simulink model "uas_main"  (R2022a)
settings: Solver=FixedStepAuto  StartTime=0.0  StopTime=10  FixedStep=sample_time  RelTol=1e-3
model workspace: external: MAT-File (data not in the file)
values from neighbouring files (symbols this model uses):
  arm_length = 0.17    [uas_trajectory.m]
  drag_coefficient = 0.47    [uas_trajectory.m]
  g = 9.80665    [uas_trajectory.m]
  inertia_xx = 0.007    [uas_trajectory.m]
  inertia_yy = 0.007    [uas_trajectory.m]
  inertia_zz = 0.012    [uas_trajectory.m]
  mass_drone = 0.68    [uas_trajectory.m]
  mass_total = mass_drone + mass_rod + mass_tip    (= 0.68)    [uas_trajectory.m]
  max_rot_velocity = 838    [uas_trajectory.m]
  mix_matrix = inv(motor_constant * allocation_matrix)    [uas_trajectory.m]
  moment_constant = 0.016    [uas_trajectory.m]
  motor_constant = 8.54858e-06    [uas_trajectory.m]
  poly_traj = uas_minimum_snap(knots, order, waypoints, corridors, make_plots)    [uas_trajectory.m]
  publish_rate = 1 * sample_time    (= 0.04)    [uas_trajectory.m]
  reference_area = pi * 75e-3^2    (= 0.0176714586764)    [uas_trajectory.m]
  rotor_offset_top = 0.01    [uas_trajectory.m]
  route = [0 0 1 ; 9 0 1 ; 9 9 1]    [uas_trajectory.m]
  sample_time = 4e-2    (= 0.04)    [uas_trajectory.m]
  x0 = 36    [uas_trajectory.m]
  y0 = 80    [uas_trajectory.m]
  z0 = 1    [uas_trajectory.m]
undefined symbols (not defined in the file or in its folder): Angular, Linear, Pose, Position, quat2rotm, X, Y, Z
libraries: nesl_utility x32, sm_lib x25, robotlib x9, simulink x1, sim3dlib x1, uavsim3dlib x1, vrlib x1
(part 2 of 2)

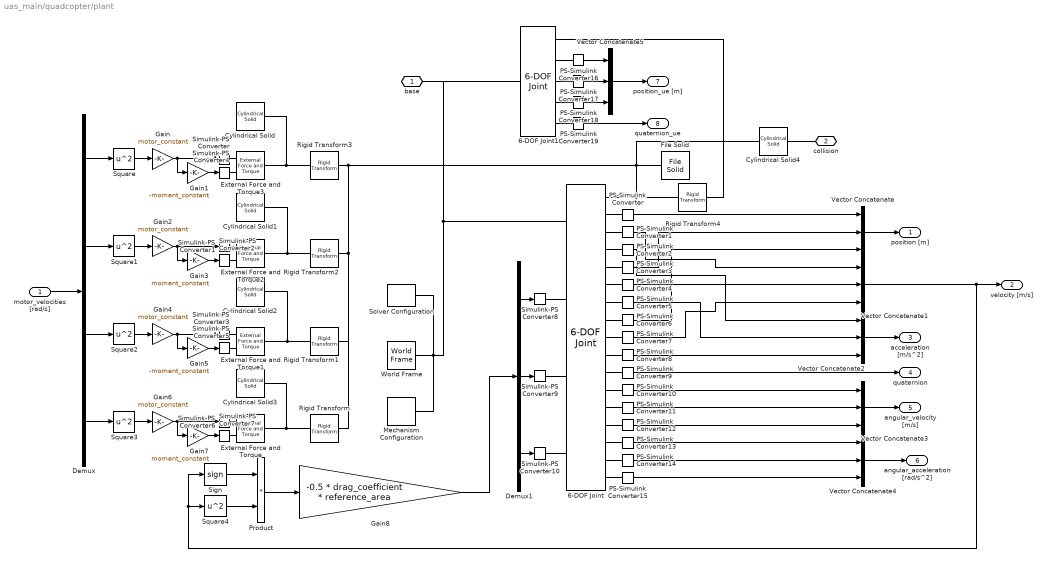
== system uas_main/quadcopter/plant ==
  motor_velocities [rad/s] : Inport
  6-DOF Joint : sm_lib/Joints/6-DOF Joint  JointMode=Normal  SenseConstraintForce=off  SenseConstraintForceX=off  SenseConstraintForceY=off  SenseConstraintForceZ=off  SenseConstraintTorque=off  SenseConstraintTorqueX=off  SenseConstraintTorqueY=off  SenseConstraintTorqueZ=off  SenseTotalForce=off  SenseTotalForceX=off  SenseTotalForceY=off  SenseTotalForceZ=off  SenseTotalTorque=off  SenseTotalTorqueX=off  SenseTotalTorqueY=off  SenseTotalTorqueZ=off  CompositeWrenchDir=BaseOnFollower  CompositeWrenchFrame=BaseFrame  PxEquilibriumPosition=0  PxEquilibriumPositionUnits=m  PxSpringStiffness=0  PxSpringStiffnessUnits=N/m  PxDampingCoefficient=0  PxDampingCoefficientUnits=N/(m/s)  PxTorqueActuationMode=InputTorque  PxMotionActuationMode=ComputedMotion  PxSensePosition=on  PxSenseVelocity=on  PxSenseAcceleration=on  PxSenseTorqueForce=off  PxSenseLowerLimitTorqueForce=off  PxSenseUpperLimitTorqueForce=off  PxLowerLimitSpecify=off  PxLowerLimitBound=-1  PxLowerLimitBoundUnits=m  PxLowerLimitStiffness=1e6  PxLowerLimitStiffnessUnits=N/m  PxLowerLimitDamping=1e3  PxLowerLimitDampingUnits=N/(m/s)  PxLowerLimitTransitionRegionWidth=1e-4  PxLowerLimitTransitionRegionWidthUnits=m  PxUpperLimitSpecify=off  PxUpperLimitBound=1  PxUpperLimitBoundUnits=m  PxUpperLimitStiffness=1e6  PxUpperLimitStiffnessUnits=N/m  PxUpperLimitDamping=1e3  PxUpperLimitDampingUnits=N/(m/s)  PxUpperLimitTransitionRegionWidth=1e-4  PxUpperLimitTransitionRegionWidthUnits=m  PxPositionTargetSpecify=on  PxPositionTargetPriority=High  PxPositionTargetValue=0  PxPositionTargetValueUnits=m  PxVelocityTargetSpecify=off  PxVelocityTargetPriority=High  PxVelocityTargetValue=0  PxVelocityTargetValueUnits=m/s  PyEquilibriumPosition=0  PyEquilibriumPositionUnits=m  PySpringStiffness=0  PySpringStiffnessUnits=N/m  PyDampingCoefficient=0  PyDampingCoefficientUnits=N/(m/s)  PyTorqueActuationMode=InputTorque  PyMotionActuationMode=ComputedMotion  PySensePosition=on  PySenseVelocity=on  PySenseAcceleration=on  PySenseTorqueForce=off  PySenseLowerLimitTorqueForce=off  PySenseUpperLimitTorqueForce=off  PyLowerLimitSpecify=off  PyLowerLimitBound=-1  PyLowerLimitBoundUnits=m  PyLowerLimitStiffness=1e6  PyLowerLimitStiffnessUnits=N/m  PyLowerLimitDamping=1e3  PyLowerLimitDampingUnits=N/(m/s)  PyLowerLimitTransitionRegionWidth=1e-4  PyLowerLimitTransitionRegionWidthUnits=m  PyUpperLimitSpecify=off  PyUpperLimitBound=1  PyUpperLimitBoundUnits=m  PyUpperLimitStiffness=1e6  PyUpperLimitStiffnessUnits=N/m  PyUpperLimitDamping=1e3  PyUpperLimitDampingUnits=N/(m/s)  PyUpperLimitTransitionRegionWidth=1e-4  PyUpperLimitTransitionRegionWidthUnits=m  PyPositionTargetSpecify=on  PyPositionTargetPriority=High  PyPositionTargetValue=0  PyPositionTargetValueUnits=m  PyVelocityTargetSpecify=off  PyVelocityTargetPriority=High  PyVelocityTargetValue=0  PyVelocityTargetValueUnits=m/s  PzEquilibriumPosition=0  PzEquilibriumPositionUnits=m  PzSpringStiffness=0  PzSpringStiffnessUnits=N/m  PzDampingCoefficient=0  PzDampingCoefficientUnits=N/(m/s)  PzTorqueActuationMode=InputTorque  PzMotionActuationMode=ComputedMotion  PzSensePosition=on  PzSenseVelocity=on  PzSenseAcceleration=on  PzSenseTorqueForce=off  PzSenseLowerLimitTorqueForce=off  PzSenseUpperLimitTorqueForce=off  PzLowerLimitSpecify=off  PzLowerLimitBound=-1  PzLowerLimitBoundUnits=m  PzLowerLimitStiffness=1e6  PzLowerLimitStiffnessUnits=N/m  PzLowerLimitDamping=1e3  PzLowerLimitDampingUnits=N/(m/s)  PzLowerLimitTransitionRegionWidth=1e-4  PzLowerLimitTransitionRegionWidthUnits=m  PzUpperLimitSpecify=off  PzUpperLimitBound=1  PzUpperLimitBoundUnits=m  PzUpperLimitStiffness=1e6  PzUpperLimitStiffnessUnits=N/m  PzUpperLimitDamping=1e3  PzUpperLimitDampingUnits=N/(m/s)  PzUpperLimitTransitionRegionWidth=1e-4  PzUpperLimitTransitionRegionWidthUnits=m  PzPositionTargetSpecify=on  PzPositionTargetPriority=High  PzPositionTargetValue=z0  PzPositionTargetValueUnits=m  PzVelocityTargetSpecify=off  PzVelocityTargetPriority=High  PzVelocityTargetValue=0  PzVelocityTargetValueUnits=m/s  SphDefPosRotationMethod=None  SphDefPosRotationAngleUnits=deg  SphDefPosRotationStandardAxis=+Z  SphDefPosRotationAngle=0.0  SphDefPosRotationArbitraryAxis=[0 0 1]  SphDefPosFollAlignAxisA=+X  SphDefPosBaseAlignAxisA=+Y  SphDefPosFollAlignAxisB=+Y  SphDefPosBaseAlignAxisB=+Z  SphDefPosRotationSequenceAxes=FollowerAxes  SphDefPosRotationSequence=XYX  SphDefPosRotationSequenceAngles=[0 0 0]  SphDefPosRotationSequenceAnglesUnits=deg  SphDefPosRotationMatrix=[1 0 0; 0 1 0; 0 0 1]  SphEqPosRotationMethod=None  SphEqPosRotationAngleUnits=deg  SphEqPosRotationStandardAxis=+Z  SphEqPosRotationAngle=0.0  SphEqPosRotationArbitraryAxis=[0 0 1]  SphEqPosFollAlignAxisA=+X  SphEqPosBaseAlignAxisA=+Y  SphEqPosFollAlignAxisB=+Y  SphEqPosBaseAlignAxisB=+Z  SphEqPosRotationSequenceAxes=FollowerAxes  SphEqPosRotationSequence=XYX  SphEqPosRotationSequenceAngles=[0 0 0]  SphEqPosRotationSequenceAnglesUnits=deg  SphEqPosRotationMatrix=[1 0 0; 0 1 0; 0 0 1]  SphSpringStiffness=0  SphSpringStiffnessUnits=N*m/deg  SphDampingCoefficient=0  SphDampingCoefficientUnits=N*m/(deg/s)  SphActuateTorqueX=off  SphActuateTorqueY=off  SphActuateTorqueZ=off  SphActuateTorque=off  SphTorqueActuationMode=NoTorque  SphMotionActuationMode=ComputedMotion  SphActuationFrame=BaseFrame  SphSensePosition=on  SphSenseVelocityX=on  SphSenseVelocityY=on  SphSenseVelocityZ=on  SphSenseVelocity=off  SphSenseAccelerationX=on  SphSenseAccelerationY=on  SphSenseAccelerationZ=on  SphSenseAcceleration=off  SphSenseTorqueX=off  SphSenseTorqueY=off  SphSenseTorqueZ=off  SphSenseTorqueForce=off  SphSenseLowerLimitTorqueMag=off  SphSenseUpperLimitTorqueMag=off  SphSensingFrame=BaseFrame  SphLowerLimitSpecify=off  SphLowerLimitBound=15  SphLowerLimitBoundUnits=deg  SphLowerLimitStiffness=1e4  SphLowerLimitStiffnessUnits=N*m/deg  SphLowerLimitDamping=10  SphLowerLimitDampingUnits=N*m/(deg/s)  SphLowerLimitTransitionRegionWidth=0.1  SphLowerLimitTransitionRegionWidthUnits=deg  SphUpperLimitSpecify=off  SphUpperLimitBound=45  SphUpperLimitBoundUnits=deg  SphUpperLimitStiffness=1e4  SphUpperLimitStiffnessUnits=N*m/deg  SphUpperLimitDamping=10  SphUpperLimitDampingUnits=N*m/(deg/s)  SphUpperLimitTransitionRegionWidth=0.1  SphUpperLimitTransitionRegionWidthUnits=deg  SphPositionTargetRotationMethod=StandardAxis  SphPositionTargetRotationAngleUnits=deg  SphPositionTargetRotationStandardAxis=+Z  SphPositionTargetRotationAngle=0  SphPositionTargetRotationArbitraryAxis=[0 0 1]  SphPositionTargetFollAlignAxisA=+X  SphPositionTargetBaseAlignAxisA=+Y  SphPositionTargetFollAlignAxisB=+Y  SphPositionTargetBaseAlignAxisB=+Z  SphPositionTargetRotationSequenceAxes=FollowerAxes  SphPositionTargetRotationSequence=XYX  SphPositionTargetRotationSequenceAngles=[0 0 0]  SphPositionTargetRotationSequenceAnglesUnits=deg  SphPositionTargetRotationMatrix=[1 0 0; 0 1 0; 0 0 1]  SphPositionTargetSpecify=on  SphPositionTargetPriority=High  SphVelocityTargetValue=[0 0 0]  SphVelocityTargetValueUnits=deg/s  SphVelocityTargetSpecify=off  SphVelocityTargetPriority=High  SphVelocityTargetInFollowerFrame=on
  6-DOF Joint1 : sm_lib/Joints/6-DOF Joint  JointMode=Normal  SenseConstraintForce=off  SenseConstraintForceX=off  SenseConstraintForceY=off  SenseConstraintForceZ=off  SenseConstraintTorque=off  SenseConstraintTorqueX=off  SenseConstraintTorqueY=off  SenseConstraintTorqueZ=off  SenseTotalForce=off  SenseTotalForceX=off  SenseTotalForceY=off  SenseTotalForceZ=off  SenseTotalTorque=off  SenseTotalTorqueX=off  SenseTotalTorqueY=off  SenseTotalTorqueZ=off  CompositeWrenchDir=FollowerOnBase  CompositeWrenchFrame=BaseFrame  PxEquilibriumPosition=0  PxEquilibriumPositionUnits=m  PxSpringStiffness=0  PxSpringStiffnessUnits=N/m  PxDampingCoefficient=0  PxDampingCoefficientUnits=N/(m/s)  PxTorqueActuationMode=NoTorque  PxMotionActuationMode=ComputedMotion  PxSensePosition=on  PxSenseVelocity=off  PxSenseAcceleration=off  PxSenseTorqueForce=off  PxSenseLowerLimitTorqueForce=off  PxSenseUpperLimitTorqueForce=off  PxLowerLimitSpecify=off  PxLowerLimitBound=-1  PxLowerLimitBoundUnits=m  PxLowerLimitStiffness=1e6  PxLowerLimitStiffnessUnits=N/m  PxLowerLimitDamping=1e3  PxLowerLimitDampingUnits=N/(m/s)  PxLowerLimitTransitionRegionWidth=1e-4  PxLowerLimitTransitionRegionWidthUnits=m  PxUpperLimitSpecify=off  PxUpperLimitBound=1  PxUpperLimitBoundUnits=m  PxUpperLimitStiffness=1e6  PxUpperLimitStiffnessUnits=N/m  PxUpperLimitDamping=1e3  PxUpperLimitDampingUnits=N/(m/s)  PxUpperLimitTransitionRegionWidth=1e-4  PxUpperLimitTransitionRegionWidthUnits=m  PxPositionTargetSpecify=off  PxPositionTargetPriority=High  PxPositionTargetValue=0  PxPositionTargetValueUnits=m  PxVelocityTargetSpecify=off  PxVelocityTargetPriority=High  PxVelocityTargetValue=0  PxVelocityTargetValueUnits=m/s  PyEquilibriumPosition=0  PyEquilibriumPositionUnits=m  PySpringStiffness=0  PySpringStiffnessUnits=N/m  PyDampingCoefficient=0  PyDampingCoefficientUnits=N/(m/s)  PyTorqueActuationMode=NoTorque  PyMotionActuationMode=ComputedMotion  PySensePosition=on  PySenseVelocity=off  PySenseAcceleration=off  PySenseTorqueForce=off  PySenseLowerLimitTorqueForce=off  PySenseUpperLimitTorqueForce=off  PyLowerLimitSpecify=off  PyLowerLimitBound=-1  PyLowerLimitBoundUnits=m  PyLowerLimitStiffness=1e6  PyLowerLimitStiffnessUnits=N/m  PyLowerLimitDamping=1e3  PyLowerLimitDampingUnits=N/(m/s)  PyLowerLimitTransitionRegionWidth=1e-4  PyLowerLimitTransitionRegionWidthUnits=m  PyUpperLimitSpecify=off  PyUpperLimitBound=1  PyUpperLimitBoundUnits=m  PyUpperLimitStiffness=1e6  PyUpperLimitStiffnessUnits=N/m  PyUpperLimitDamping=1e3  PyUpperLimitDampingUnits=N/(m/s)  PyUpperLimitTransitionRegionWidth=1e-4  PyUpperLimitTransitionRegionWidthUnits=m  PyPositionTargetSpecify=off  PyPositionTargetPriority=High  PyPositionTargetValue=0  PyPositionTargetValueUnits=m  PyVelocityTargetSpecify=off  PyVelocityTargetPriority=High  PyVelocityTargetValue=0  PyVelocityTargetValueUnits=m/s  PzEquilibriumPosition=0  PzEquilibriumPositionUnits=m  PzSpringStiffness=0  PzSpringStiffnessUnits=N/m  PzDampingCoefficient=0  PzDampingCoefficientUnits=N/(m/s)  PzTorqueActuationMode=NoTorque  PzMotionActuationMode=ComputedMotion  PzSensePosition=on  PzSenseVelocity=off  PzSenseAcceleration=off  PzSenseTorqueForce=off  PzSenseLowerLimitTorqueForce=off  PzSenseUpperLimitTorqueForce=off  PzLowerLimitSpecify=off  PzLowerLimitBound=-1  PzLowerLimitBoundUnits=m  PzLowerLimitStiffness=1e6  PzLowerLimitStiffnessUnits=N/m  PzLowerLimitDamping=1e3  PzLowerLimitDampingUnits=N/(m/s)  PzLowerLimitTransitionRegionWidth=1e-4  PzLowerLimitTransitionRegionWidthUnits=m  PzUpperLimitSpecify=off  PzUpperLimitBound=1  PzUpperLimitBoundUnits=m  PzUpperLimitStiffness=1e6  PzUpperLimitStiffnessUnits=N/m  PzUpperLimitDamping=1e3  PzUpperLimitDampingUnits=N/(m/s)  PzUpperLimitTransitionRegionWidth=1e-4  PzUpperLimitTransitionRegionWidthUnits=m  PzPositionTargetSpecify=off  PzPositionTargetPriority=High  PzPositionTargetValue=0  PzPositionTargetValueUnits=m  PzVelocityTargetSpecify=off  PzVelocityTargetPriority=High  PzVelocityTargetValue=0  PzVelocityTargetValueUnits=m/s  SphDefPosRotationMethod=None  SphDefPosRotationAngleUnits=deg  SphDefPosRotationStandardAxis=+Z  SphDefPosRotationAngle=0.0  SphDefPosRotationArbitraryAxis=[0 0 1]  SphDefPosFollAlignAxisA=+X  SphDefPosBaseAlignAxisA=+Y  SphDefPosFollAlignAxisB=+Y  SphDefPosBaseAlignAxisB=+Z  SphDefPosRotationSequenceAxes=FollowerAxes  SphDefPosRotationSequence=XYX  SphDefPosRotationSequenceAngles=[0 0 0]  SphDefPosRotationSequenceAnglesUnits=deg  SphDefPosRotationMatrix=[1 0 0; 0 1 0; 0 0 1]  SphEqPosRotationMethod=None  SphEqPosRotationAngleUnits=deg  SphEqPosRotationStandardAxis=+Z  SphEqPosRotationAngle=0.0  SphEqPosRotationArbitraryAxis=[0 0 1]  SphEqPosFollAlignAxisA=+X  SphEqPosBaseAlignAxisA=+Y  SphEqPosFollAlignAxisB=+Y  SphEqPosBaseAlignAxisB=+Z  SphEqPosRotationSequenceAxes=FollowerAxes  SphEqPosRotationSequence=XYX  SphEqPosRotationSequenceAngles=[0 0 0]  SphEqPosRotationSequenceAnglesUnits=deg  SphEqPosRotationMatrix=[1 0 0; 0 1 0; 0 0 1]  SphSpringStiffness=0  SphSpringStiffnessUnits=N*m/deg  SphDampingCoefficient=0  SphDampingCoefficientUnits=N*m/(deg/s)  SphActuateTorqueX=off  SphActuateTorqueY=off  SphActuateTorqueZ=off  SphActuateTorque=off  SphTorqueActuationMode=NoTorque  SphMotionActuationMode=ComputedMotion  SphActuationFrame=BaseFrame  SphSensePosition=on  SphSenseVelocityX=off  SphSenseVelocityY=off  SphSenseVelocityZ=off  SphSenseVelocity=off  SphSenseAccelerationX=off  SphSenseAccelerationY=off  SphSenseAccelerationZ=off  SphSenseAcceleration=off  SphSenseTorqueX=off  SphSenseTorqueY=off  SphSenseTorqueZ=off  SphSenseTorqueForce=off  SphSenseLowerLimitTorqueMag=off  SphSenseUpperLimitTorqueMag=off  SphSensingFrame=BaseFrame  SphLowerLimitSpecify=off  SphLowerLimitBound=15  SphLowerLimitBoundUnits=deg  SphLowerLimitStiffness=1e4  SphLowerLimitStiffnessUnits=N*m/deg  SphLowerLimitDamping=10  SphLowerLimitDampingUnits=N*m/(deg/s)  SphLowerLimitTransitionRegionWidth=0.1  SphLowerLimitTransitionRegionWidthUnits=deg  SphUpperLimitSpecify=off  SphUpperLimitBound=45  SphUpperLimitBoundUnits=deg  SphUpperLimitStiffness=1e4  SphUpperLimitStiffnessUnits=N*m/deg  SphUpperLimitDamping=10  SphUpperLimitDampingUnits=N*m/(deg/s)  SphUpperLimitTransitionRegionWidth=0.1  SphUpperLimitTransitionRegionWidthUnits=deg  SphPositionTargetRotationMethod=None  SphPositionTargetRotationAngleUnits=deg  SphPositionTargetRotationStandardAxis=+Z  SphPositionTargetRotationAngle=0.0  SphPositionTargetRotationArbitraryAxis=[0 0 1]  SphPositionTargetFollAlignAxisA=+X  SphPositionTargetBaseAlignAxisA=+Y  SphPositionTargetFollAlignAxisB=+Y  SphPositionTargetBaseAlignAxisB=+Z  SphPositionTargetRotationSequenceAxes=FollowerAxes  SphPositionTargetRotationSequence=XYX  SphPositionTargetRotationSequenceAngles=[0 0 0]  SphPositionTargetRotationSequenceAnglesUnits=deg  SphPositionTargetRotationMatrix=[1 0 0; 0 1 0; 0 0 1]  SphPositionTargetSpecify=off  SphPositionTargetPriority=High  SphVelocityTargetValue=[0 0 0]  SphVelocityTargetValueUnits=deg/s  SphVelocityTargetSpecify=off  SphVelocityTargetPriority=High  SphVelocityTargetInFollowerFrame=on
  Cylindrical Solid : sm_lib/Body Elements/Cylindrical Solid  GraphicAmbientColor=[0.15 0.15 0.15 1.0]  BasedOnType=Density  CenterOfMass=[0 0 0]  CenterOfMassUnits=m  GraphicDiffuseColor=[1.0 0.0 0.0]  CylinderLength=1  CylinderLengthUnits=mm  CylinderRadius=100  CylinderRadiusUnits=mm  Density=0  DensityUnits=kg/m^3  DoExposeReferenceFrame=on  GraphicEmissiveColor=[0.0 0.0 0.0 1.0]  ExportEntireGeometry=off  SerializedFrames=<Frames/>  MarkerShape=Sphere  MarkerSize=10  GraphicType=FromGeometry  InertiaType=CalculateFromGeometry  Mass=1  MassUnits=kg  MomentsOfInertia=[1 1 1]  MomentsOfInertiaUnits=kg*m^2  GraphicOpacity=0.5  ProductsOfInertia=[0 0 0]  ProductsOfInertiaUnits=kg*m^2  GraphicShininess=75  GraphicSpecularColor=[0.5 0.5 0.5 1.0]  GraphicVisPropType=SimpleVisualProperties
  Cylindrical Solid1 : sm_lib/Body Elements/Cylindrical Solid  GraphicAmbientColor=[0.15 0.15 0.15 1.0]  BasedOnType=Density  CenterOfMass=[0 0 0]  CenterOfMassUnits=m  GraphicDiffuseColor=[0 1 0]  CylinderLength=1  CylinderLengthUnits=mm  CylinderRadius=100  CylinderRadiusUnits=mm  Density=0  DensityUnits=kg/m^3  DoExposeReferenceFrame=on  GraphicEmissiveColor=[0.0 0.0 0.0 1.0]  ExportEntireGeometry=off  SerializedFrames=<Frames/>  MarkerShape=Sphere  MarkerSize=10  GraphicType=FromGeometry  InertiaType=CalculateFromGeometry  Mass=1  MassUnits=kg  MomentsOfInertia=[1 1 1]  MomentsOfInertiaUnits=kg*m^2  GraphicOpacity=0.5  ProductsOfInertia=[0 0 0]  ProductsOfInertiaUnits=kg*m^2  GraphicShininess=75  GraphicSpecularColor=[0.5 0.5 0.5 1.0]  GraphicVisPropType=SimpleVisualProperties
  Cylindrical Solid2 : sm_lib/Body Elements/Cylindrical Solid  GraphicAmbientColor=[0.15 0.15 0.15 1.0]  BasedOnType=Density  CenterOfMass=[0 0 0]  CenterOfMassUnits=m  GraphicDiffuseColor=[0 0 1]  CylinderLength=1  CylinderLengthUnits=mm  CylinderRadius=100  CylinderRadiusUnits=mm  Density=0  DensityUnits=kg/m^3  DoExposeReferenceFrame=on  GraphicEmissiveColor=[0.0 0.0 0.0 1.0]  ExportEntireGeometry=off  SerializedFrames=<Frames/>  MarkerShape=Sphere  MarkerSize=10  GraphicType=FromGeometry  InertiaType=CalculateFromGeometry  Mass=1  MassUnits=kg  MomentsOfInertia=[1 1 1]  MomentsOfInertiaUnits=kg*m^2  GraphicOpacity=0.5  ProductsOfInertia=[0 0 0]  ProductsOfInertiaUnits=kg*m^2  GraphicShininess=75  GraphicSpecularColor=[0.5 0.5 0.5 1.0]  GraphicVisPropType=SimpleVisualProperties
  Cylindrical Solid3 : sm_lib/Body Elements/Cylindrical Solid  GraphicAmbientColor=[0.15 0.15 0.15 1.0]  BasedOnType=Density  CenterOfMass=[0 0 0]  CenterOfMassUnits=m  GraphicDiffuseColor=[0 0 1]  CylinderLength=1  CylinderLengthUnits=mm  CylinderRadius=100  CylinderRadiusUnits=mm  Density=0  DensityUnits=kg/m^3  DoExposeReferenceFrame=on  GraphicEmissiveColor=[0.0 0.0 0.0 1.0]  ExportEntireGeometry=off  SerializedFrames=<Frames/>  MarkerShape=Sphere  MarkerSize=10  GraphicType=FromGeometry  InertiaType=CalculateFromGeometry  Mass=1  MassUnits=kg  MomentsOfInertia=[1 1 1]  MomentsOfInertiaUnits=kg*m^2  GraphicOpacity=0.5  ProductsOfInertia=[0 0 0]  ProductsOfInertiaUnits=kg*m^2  GraphicShininess=75  GraphicSpecularColor=[0.5 0.5 0.5 1.0]  GraphicVisPropType=SimpleVisualProperties
  Cylindrical Solid4 : sm_lib/Body Elements/Cylindrical Solid  GraphicAmbientColor=[0.15 0.15 0.15 1.0]  BasedOnType=Density  CenterOfMass=[0 0 0]  CenterOfMassUnits=m  GraphicDiffuseColor=[0.5 0.5 0.5]  CylinderLength=0.3  CylinderLengthUnits=m  CylinderRadius=0.27  CylinderRadiusUnits=m  Density=0  DensityUnits=kg/m^3  DoExposeReferenceFrame=on  GraphicEmissiveColor=[0.0 0.0 0.0 1.0]  ExportEntireGeometry=on  SerializedFrames=<Frames/>  MarkerShape=Sphere  MarkerSize=10  GraphicType=FromGeometry  InertiaType=CalculateFromGeometry  Mass=1  MassUnits=kg  MomentsOfInertia=[1 1 1]  MomentsOfInertiaUnits=kg*m^2  GraphicOpacity=0.2  ProductsOfInertia=[0 0 0]  ProductsOfInertiaUnits=kg*m^2  GraphicShininess=75  GraphicSpecularColor=[0.5 0.5 0.5 1.0]  GraphicVisPropType=SimpleVisualProperties
  Demux : Demux
  Demux1 : Demux  Outputs=3
  External Force and Torque{,1..3} (4 alike) : sm_lib/Forces and Torques/External Force and Torque  ForceResolutionFrame=AttachedFrame  EnableForceX=off  EnableForceY=off  EnableForceZ=on  EnableForce=off  TorqueResolutionFrame=AttachedFrame  EnableTorqueX=off  EnableTorqueY=off  EnableTorqueZ=on  EnableTorque=off
  File Solid : sm_lib/Body Elements/File Solid  ExtGeomFileName=uas_geometry.stl  UnitType=Custom  ExtGeomFileUnits=m  StepReaderType=HEX  ExportConvexHullGeometry=off  InertiaType=Custom  Mass=mass_drone  MassUnits=kg  CenterOfMass=[0 0 0]  CenterOfMassUnits=m  MomentsOfInertia=[inertia_xx inertia_yy inertia_zz]  MomentsOfInertiaUnits=kg*m^2  ProductsOfInertia=[0 0 0]  ProductsOfInertiaUnits=kg*m^2  BasedOnType=DensityFromFile  Density=1000  DensityUnits=kg/m^3  DoExposeReferenceFrame=on  SerializedFrames=<Frames/>  GraphicType=FromGeometry  MarkerShape=Sphere  MarkerSize=10  GraphicVisPropType=SimpleVisualProperties  GraphicDiffuseColor=[1.0 1.0 1.0]  GraphicSpecularColor=[0.5 0.5 0.5 1.0]  GraphicAmbientColor=[0.15 0.15 0.15 1.0]  GraphicEmissiveColor=[0.0 0.0 0.0 1.0]  GraphicShininess=75  GraphicOpacity=1.0
  Gain{,2,4,6} (4 alike) : Gain  Gain=motor_constant
  Gain1 : Gain  Gain=-moment_constant
  Gain3 : Gain  Gain=moment_constant
  Gain5 : Gain  Gain=-moment_constant
  Gain7 : Gain  Gain=moment_constant
  Gain8 : Gain  Gain=-0.5 * drag_coefficient * reference_area
  Mechanism Configuration : sm_lib/Utilities/Mechanism Configuration  UniformGravity=Constant  GravityVector=[0 0 -9.80665]  GravityUnits=m/s^2  LinearizationDelta=0.001  JointModeTransitionNonlinearIterations=2
  PS-Simulink Converter{,1..19} (20 alike) : nesl_utility/PS-Simulink Converter  PhysicalDomain=network_engine_domain  SubClassName=ps_output  LeftPortType=input  RightPortType=output  PseudoPeriodic=off  Frequencies=[]  VectorFormat=1-D array  Unit=inherit  AffineConversion=off
      settings: SourceProductBaseCode=SS,PW,VE
  Product : Product
  Rigid Transform : sm_lib/Frames and Transforms/Rigid Transform  TranslationMethod=Cartesian  TranslationStandardOffset=0  TranslationLengthUnit=m  TranslationStandardAxis=+Z  TranslationCartesianOffset=[0 -arm_length rotor_offset_top]  TranslationROffset=0  TranslationROffsetUnits=m  TranslationZOffset=0  TranslationZOffsetUnits=m  TranslationThetaOffset=0  TranslationThetaOffsetUnits=deg  RotationMethod=None  RotationAngleUnits=deg  RotationStandardAxis=+Z  RotationAngle=0.0  RotationArbitraryAxis=[0 0 1]  FollAlignAxisA=+X  BaseAlignAxisA=+Y  FollAlignAxisB=+Y  BaseAlignAxisB=+Z  RotationSequenceAxes=FollowerAxes  RotationSequence=XYX  RotationSequenceAngles=[0 0 0]  RotationSequenceAnglesUnits=deg  RotationMatrix=[1 0 0; 0 1 0; 0 0 1]
  Rigid Transform1 : sm_lib/Frames and Transforms/Rigid Transform  TranslationMethod=Cartesian  TranslationStandardOffset=0  TranslationLengthUnit=m  TranslationStandardAxis=+Z  TranslationCartesianOffset=[-arm_length 0 rotor_offset_top]  TranslationROffset=0  TranslationROffsetUnits=m  TranslationZOffset=0  TranslationZOffsetUnits=m  TranslationThetaOffset=0  TranslationThetaOffsetUnits=deg  RotationMethod=None  RotationAngleUnits=deg  RotationStandardAxis=+Z  RotationAngle=0.0  RotationArbitraryAxis=[0 0 1]  FollAlignAxisA=+X  BaseAlignAxisA=+Y  FollAlignAxisB=+Y  BaseAlignAxisB=+Z  RotationSequenceAxes=FollowerAxes  RotationSequence=XYX  RotationSequenceAngles=[0 0 0]  RotationSequenceAnglesUnits=deg  RotationMatrix=[1 0 0; 0 1 0; 0 0 1]
  Rigid Transform2 : sm_lib/Frames and Transforms/Rigid Transform  TranslationMethod=Cartesian  TranslationStandardOffset=0  TranslationLengthUnit=m  TranslationStandardAxis=+Z  TranslationCartesianOffset=[0 arm_length rotor_offset_top]  TranslationROffset=0  TranslationROffsetUnits=m  TranslationZOffset=0  TranslationZOffsetUnits=m  TranslationThetaOffset=0  TranslationThetaOffsetUnits=deg  RotationMethod=None  RotationAngleUnits=deg  RotationStandardAxis=+Z  RotationAngle=0.0  RotationArbitraryAxis=[0 0 1]  FollAlignAxisA=+X  BaseAlignAxisA=+Y  FollAlignAxisB=+Y  BaseAlignAxisB=+Z  RotationSequenceAxes=FollowerAxes  RotationSequence=XYX  RotationSequenceAngles=[0 0 0]  RotationSequenceAnglesUnits=deg  RotationMatrix=[1 0 0; 0 1 0; 0 0 1]
  Rigid Transform3 : sm_lib/Frames and Transforms/Rigid Transform  TranslationMethod=Cartesian  TranslationStandardOffset=0  TranslationLengthUnit=m  TranslationStandardAxis=+Z  TranslationCartesianOffset=[arm_length 0 rotor_offset_top]  TranslationROffset=0  TranslationROffsetUnits=m  TranslationZOffset=0  TranslationZOffsetUnits=m  TranslationThetaOffset=0  TranslationThetaOffsetUnits=deg  RotationMethod=None  RotationAngleUnits=deg  RotationStandardAxis=+Z  RotationAngle=0.0  RotationArbitraryAxis=[0 0 1]  FollAlignAxisA=+X  BaseAlignAxisA=+Y  FollAlignAxisB=+Y  BaseAlignAxisB=+Z  RotationSequenceAxes=FollowerAxes  RotationSequence=XYX  RotationSequenceAngles=[0 0 0]  RotationSequenceAnglesUnits=deg  RotationMatrix=[1 0 0; 0 1 0; 0 0 1]
  Rigid Transform4 : sm_lib/Frames and Transforms/Rigid Transform  TranslationMethod=StandardAxis  TranslationStandardOffset=0.15  TranslationLengthUnit=m  TranslationStandardAxis=-Z  TranslationCartesianOffset=[0 0 0]  TranslationROffset=0  TranslationROffsetUnits=m  TranslationZOffset=0  TranslationZOffsetUnits=m  TranslationThetaOffset=0  TranslationThetaOffsetUnits=deg  RotationMethod=None  RotationAngleUnits=deg  RotationStandardAxis=+Z  RotationAngle=0.0  RotationArbitraryAxis=[0 0 1]  FollAlignAxisA=+X  BaseAlignAxisA=+Y  FollAlignAxisB=+Y  BaseAlignAxisB=+Z  RotationSequenceAxes=FollowerAxes  RotationSequence=XYX  RotationSequenceAngles=[0 0 0]  RotationSequenceAnglesUnits=deg  RotationMatrix=[1 0 0; 0 1 0; 0 0 1]
  Sign : Signum
  Simulink-PS Converter{,1..10} (11 alike) : nesl_utility/Simulink-PS Converter  PhysicalDomain=network_engine_domain  SubClassName=ps_input  LeftPortType=input  RightPortType=output  PseudoPeriodic=off  Frequencies=[]  NoiseDistribution=none  NoiseParameters=[]  Unit=1  AffineConversion=off  FilteringAndDerivatives=provide  SimscapeFilterOrder=1  InputFilterTimeConstant=0.001  UdotUserProvided=0
      settings: SourceProductBaseCode=SS,PW,VE
  Solver Configuration : nesl_utility/Solver Configuration  PhysicalDomain=network_engine_domain  SubClassName=solver  LeftPortType=input  RightPortType=generic  Tones=[]  Harmonics=[]  SimulateNoise=off  Profile=off  UseLocalSampling=off  EnableSwitchedLinearOptims=on  FrequencyDomain=off  UseCCode=off  RelTol=0.001  AbsTol=1e-06  MinStep=1e-09  ToWorkspace=off  RevertToSquareIcSolve=off  NumHomotopyIterations=100  PhasorMode=off  PhasorModeNumHarmonics=1  IndexReductionMethod=DerivativeReplacement  DoDC=off  ResidualTolerance=1e-09  UseLocalSolver=off  LocalSolverChoice=NE_BACKWARD_EULER_ADVANCER  LocalSolverSampleTime=0.001  DoFixedCost=off  MaxNonlinIter=3  MaxModeIter=2  ComputeImpulses=off  ImpulseIterations=2  LinearAlgebra=Sparse  LinearAlgebraNumThread=0  EquationFormulation=NE_TIME_EF  DelaysMemoryBudget=1024  AutomaticFiltering=on  FilteringTimeConstant=0.001  PartitionStorageMethod=AS_NEEDED  PartitionMemoryBudget=1024  PartitionMethod=FAST
      settings: SourceProductBaseCode=SS,PW,VE
  Square{,1..4} (5 alike) : Math  Operator=square
  Vector Concatenate{,1..5} (6 alike) : Concatenate  NumInputs=3  Mode=Multidimensional array
  World Frame : sm_lib/Frames and Transforms/World Frame
  base : PMIOPort  Side=Right
  collision : PMIOPort  Port=2  Side=Right
  position [m] : Outport
  velocity [m/s] : Outport  Port=2
  acceleration [m/s^2] : Outport  Port=3
  quaternion : Outport  Port=4  PortDimensions=[1 4]
  angular_velocity [m/s] : Outport  Port=5
  angular_acceleration [rad/s^2] : Outport  Port=6
  position_ue [m] : Outport  Port=7
  quaternion_ue : Outport  Port=8
  wires:
  Square/1 -> Gain/1
  Gain/1 -> Gain1/1, Simulink-PS Converter/1
  Gain1/1 -> Simulink-PS Converter4/1
  Square1/1 -> Gain2/1
  Gain2/1 -> Gain3/1, Simulink-PS Converter1/1
  Gain3/1 -> Simulink-PS Converter2/1
  Gain5/1 -> Simulink-PS Converter5/1
  Square2/1 -> Gain4/1
  Gain4/1 -> Gain5/1, Simulink-PS Converter3/1
  Gain7/1 -> Simulink-PS Converter7/1
  Square3/1 -> Gain6/1
  Gain6/1 -> Gain7/1, Simulink-PS Converter6/1
  Demux/1 -> Square/1
  Demux/2 -> Square1/1
  Demux/3 -> Square2/1
  Demux/4 -> Square3/1
  motor_velocities [rad/s]/1 -> Demux/1
  Vector Concatenate/1 -> position [m]/1
  Vector Concatenate1/1 -> velocity [m/s]/1, Sign/1, Square4/1
  Vector Concatenate2/1 -> acceleration [m/s^2]/1
  PS-Simulink Converter9/1 -> quaternion/1
  Vector Concatenate3/1 -> angular_velocity [m/s]/1
  Vector Concatenate4/1 -> angular_acceleration [rad/s^2]/1
  PS-Simulink Converter/1 -> Vector Concatenate/1
  PS-Simulink Converter3/1 -> Vector Concatenate/2
  PS-Simulink Converter6/1 -> Vector Concatenate/3
  PS-Simulink Converter1/1 -> Vector Concatenate1/1
  PS-Simulink Converter4/1 -> Vector Concatenate1/2
  PS-Simulink Converter7/1 -> Vector Concatenate1/3
  PS-Simulink Converter2/1 -> Vector Concatenate2/1
  PS-Simulink Converter5/1 -> Vector Concatenate2/2
  PS-Simulink Converter8/1 -> Vector Concatenate2/3
  PS-Simulink Converter10/1 -> Vector Concatenate3/1
  PS-Simulink Converter11/1 -> Vector Concatenate3/2
  PS-Simulink Converter12/1 -> Vector Concatenate3/3
  PS-Simulink Converter13/1 -> Vector Concatenate4/1
  PS-Simulink Converter14/1 -> Vector Concatenate4/2
  PS-Simulink Converter15/1 -> Vector Concatenate4/3
  Demux1/1 -> Simulink-PS Converter8/1
  Demux1/2 -> Simulink-PS Converter9/1
  Demux1/3 -> Simulink-PS Converter10/1
  Gain8/1 -> Demux1/1
  Vector Concatenate5/1 -> position_ue [m]/1
  PS-Simulink Converter16/1 -> Vector Concatenate5/1
  PS-Simulink Converter17/1 -> Vector Concatenate5/2
  PS-Simulink Converter18/1 -> Vector Concatenate5/3
  PS-Simulink Converter19/1 -> quaternion_ue/1
  Product/1 -> Gain8/1
  Sign/1 -> Product/1
  Square4/1 -> Product/2
  connections:
  Rigid Transform/LConn1 -- Rigid Transform1/LConn1 -- Rigid Transform2/LConn1 -- Rigid Transform3/LConn1 -- Cylindrical Solid4/RConn1 -- File Solid/RConn1 -- Rigid Transform4/LConn1 -- 6-DOF Joint/RConn1
  World Frame/RConn1 -- 6-DOF Joint1/LConn1 -- base/RConn1 -- 6-DOF Joint/LConn1 -- Mechanism Configuration/RConn1 -- Solver Configuration/RConn1
  External Force and Torque3/RConn1 -- Cylindrical Solid/RConn1 -- Rigid Transform3/RConn1
  External Force and Torque2/RConn1 -- Cylindrical Solid1/RConn1 -- Rigid Transform2/RConn1
  External Force and Torque1/RConn1 -- Cylindrical Solid2/RConn1 -- Rigid Transform1/RConn1
  External Force and Torque/RConn1 -- Cylindrical Solid3/RConn1 -- Rigid Transform/RConn1
  Simulink-PS Converter/RConn1 -- External Force and Torque3/LConn1
  Simulink-PS Converter4/RConn1 -- External Force and Torque3/LConn2
  Simulink-PS Converter1/RConn1 -- External Force and Torque2/LConn1
  Simulink-PS Converter2/RConn1 -- External Force and Torque2/LConn2
  Simulink-PS Converter3/RConn1 -- External Force and Torque1/LConn1
  Simulink-PS Converter5/RConn1 -- External Force and Torque1/LConn2
  Simulink-PS Converter6/RConn1 -- External Force and Torque/LConn1
  Simulink-PS Converter7/RConn1 -- External Force and Torque/LConn2
  PS-Simulink Converter/LConn1 -- 6-DOF Joint/RConn2
  6-DOF Joint/RConn3 -- PS-Simulink Converter1/LConn1
  6-DOF Joint/RConn4 -- PS-Simulink Converter2/LConn1
  6-DOF Joint/RConn5 -- PS-Simulink Converter3/LConn1
  PS-Simulink Converter4/LConn1 -- 6-DOF Joint/RConn6
  PS-Simulink Converter5/LConn1 -- 6-DOF Joint/RConn7
  PS-Simulink Converter6/LConn1 -- 6-DOF Joint/RConn8
  PS-Simulink Converter7/LConn1 -- 6-DOF Joint/RConn9
  6-DOF Joint/RConn11 -- PS-Simulink Converter9/LConn1
  6-DOF Joint/RConn10 -- PS-Simulink Converter8/LConn1
  6-DOF Joint/RConn17 -- PS-Simulink Converter15/LConn1
  6-DOF Joint/RConn16 -- PS-Simulink Converter14/LConn1
  6-DOF Joint/RConn15 -- PS-Simulink Converter13/LConn1
  6-DOF Joint/RConn14 -- PS-Simulink Converter12/LConn1
  6-DOF Joint/RConn13 -- PS-Simulink Converter11/LConn1
  6-DOF Joint/RConn12 -- PS-Simulink Converter10/LConn1
  Simulink-PS Converter8/RConn1 -- 6-DOF Joint/LConn2
  Simulink-PS Converter10/RConn1 -- 6-DOF Joint/LConn4
  Simulink-PS Converter9/RConn1 -- 6-DOF Joint/LConn3
  PS-Simulink Converter16/LConn1 -- 6-DOF Joint1/RConn2
  PS-Simulink Converter17/LConn1 -- 6-DOF Joint1/RConn3
  PS-Simulink Converter18/LConn1 -- 6-DOF Joint1/RConn4
  PS-Simulink Converter19/LConn1 -- 6-DOF Joint1/RConn5
  6-DOF Joint1/RConn1 -- Rigid Transform4/RConn1
  collision/RConn1 -- Cylindrical Solid4/LConn1

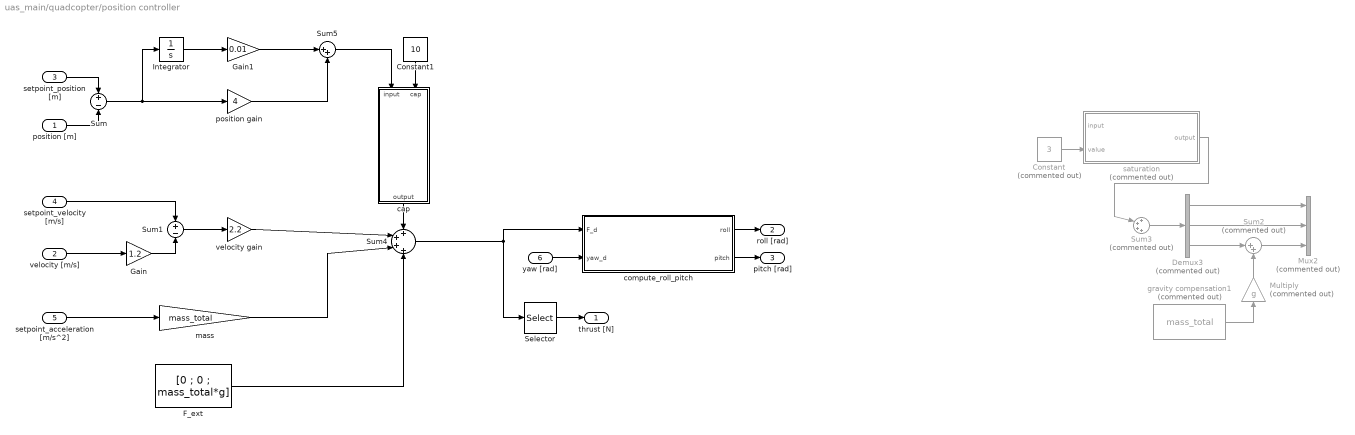
== system uas_main/quadcopter/position controller ==
  position [m] : Inport
  velocity [m/s] : Inport  Port=2
  setpoint_position [m] : Inport  Port=3
  setpoint_velocity [m/s] : Inport  Port=4
  setpoint_acceleration [m/s^2] : Inport  Port=5
  yaw [rad] : Inport  Port=6
  Constant : Constant  Commented=on  Value=3
  Constant1 : Constant  Value=10
  Demux3 : Demux  Commented=on  Outputs=3
  F_ext : Constant  Value=[0 ; 0 ; mass_total*g]  VectorParams1D=off
  Gain : Gain  Gain=1.2
  Gain1 : Gain  Gain=0.01
  Integrator : Integrator
  Multiply : Gain  Commented=on  Gain=g
  Mux2 : Mux  Commented=on  Inputs=3
  Selector : Selector  InputPortWidth=3  IndexOptions=Index vector (dialog)  Indices=[3]  OutputSizes=1
  Sum : Sum  Inputs=+|-
  Sum1 : Sum  Inputs=+|-
  Sum2 : Sum  Commented=on  Inputs=|++
  Sum3 : Sum  Commented=on  Inputs=++++
  Sum4 : Sum  Inputs=++++
  Sum5 : Sum  Inputs=|++
  cap : Subsystem
  compute_roll_pitch : MATLAB Function  TreatAsAtomicUnit=on
  gravity compensation1 : Constant  Commented=on  Value=mass_total  VectorParams1D=off
  mass : Gain  Gain=mass_total
  position gain : Gain  Gain=4
  saturation : Subsystem  Commented=on
  velocity gain : Gain  Gain=2.2
  thrust [N] : Outport
  roll [rad] : Outport  Port=2
  pitch [rad] : Outport  Port=3
  wires:
  saturation/1(output) -> Sum3/2
  gravity compensation1/1 -> Multiply/1
  Demux3/3 -> Sum2/1
  Constant/1 -> saturation/2(value)
  Sum2/1 -> Mux2/3
  Sum1/1 -> velocity gain/1
  Sum3/1 -> Demux3/1
  Demux3/1 -> Mux2/1
  Demux3/2 -> Mux2/2
  compute_roll_pitch/1(roll) -> roll [rad]/1
  Multiply/1 -> Sum2/2
  setpoint_position [m]/1 -> Sum/1
  compute_roll_pitch/2(pitch) -> pitch [rad]/1
  position [m]/1 -> Sum/2
  yaw [rad]/1 -> compute_roll_pitch/2(yaw_d)
  setpoint_velocity [m/s]/1 -> Sum1/1
  Sum/1 -> Integrator/1, position gain/1
  velocity [m/s]/1 -> Gain/1
  Gain/1 -> Sum1/2
  Integrator/1 -> Gain1/1
  setpoint_acceleration [m/s^2]/1 -> mass/1
  Gain1/1 -> Sum5/1
  position gain/1 -> Sum5/2
  velocity gain/1 -> Sum4/2
  mass/1 -> Sum4/3
  Sum4/1 -> compute_roll_pitch/1(F_d), Selector/1
  Selector/1 -> thrust [N]/1
  F_ext/1 -> Sum4/4
  cap/1(output) -> Sum4/1
  Sum5/1 -> cap/1(input)
  Constant1/1 -> cap/2(cap)

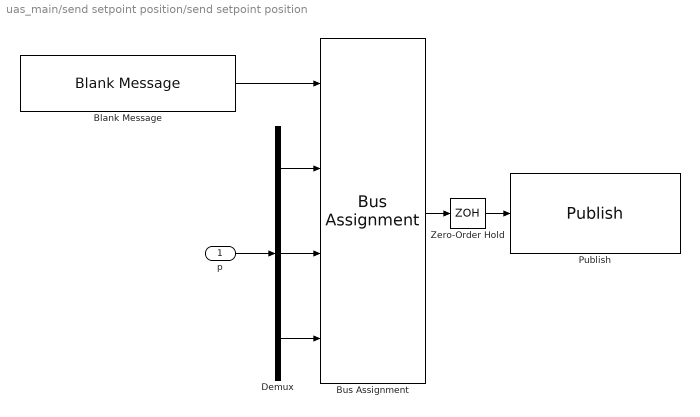
== system uas_main/send setpoint position/send setpoint position ==
  p : Inport
  Blank Message : robotlib/Blank Message  messageClass=Message  entityType=geometry_msgs/Pose  messageType=geometry_msgs/Pose  SampleTime=inf  legacyBusStruct=off
  Bus Assignment : BusAssignment  AssignedSignals=Position.X,Position.Y,Position.Z
  Demux : Demux  Outputs=3
  Publish : robotlib/Publish  topicSource=Select from ROS network  topic=/crazyflie/cmd_position  messageType=geometry_msgs/Pose  legacyBusStruct=off  messageQueueLength=1
  Zero-Order Hold : ZeroOrderHold  SampleTime=publish_rate
  wires:
  Bus Assignment/1 -> Zero-Order Hold/1
  Blank Message/1 -> Bus Assignment/1
  Zero-Order Hold/1 -> Publish/1
  Demux/1 -> Bus Assignment/2
  Demux/2 -> Bus Assignment/3
  Demux/3 -> Bus Assignment/4
  p/1 -> Demux/1

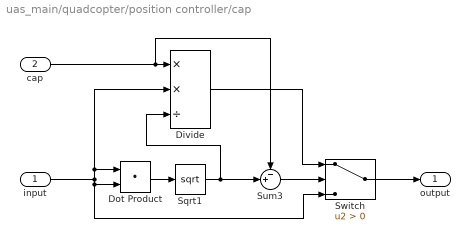
== system uas_main/quadcopter/position controller/cap ==
  input : Inport
  cap : Inport  Port=2
  Divide : Product  Inputs=**/
  Dot Product : DotProduct  OutDataTypeStr=Inherit: Inherit via internal rule
  Sqrt1 : Sqrt
  Sum3 : Sum  Inputs=-+|
  Switch : Switch  Criteria=u2 > Threshold  SaturateOnIntegerOverflow=off  InputSameDT=off
  output : Outport
  wires:
  Divide/1 -> Switch/1
  cap/1 -> Divide/1, Sum3/1
  Dot Product/1 -> Sqrt1/1
  Switch/1 -> output/1
  Sum3/1 -> Switch/2
  input/1 -> Switch/3, Dot Product/2, Divide/2, Dot Product/1
  Sqrt1/1 -> Sum3/2, Divide/3

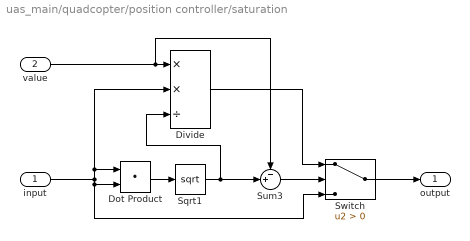
== system uas_main/quadcopter/position controller/saturation ==
  input : Inport
  value : Inport  Port=2
  Divide : Product  Inputs=**/
  Dot Product : DotProduct  OutDataTypeStr=Inherit: Inherit via internal rule
  Sqrt1 : Sqrt
  Sum3 : Sum  Inputs=-+|
  Switch : Switch  Criteria=u2 > Threshold  SaturateOnIntegerOverflow=off  InputSameDT=off
  output : Outport
  wires:
  Divide/1 -> Switch/1
  value/1 -> Divide/1, Sum3/1
  Dot Product/1 -> Sqrt1/1
  Switch/1 -> output/1
  Sum3/1 -> Switch/2
  input/1 -> Switch/3, Dot Product/2, Divide/2, Dot Product/1
  Sqrt1/1 -> Sum3/2, Divide/3

== matlab function uas_main/quadcopter/Subsystem/MATLAB Function1 ==
  data: roll input size=1; pitch input size=1; yaw input size=1; er output size=[3 1]; R input size=[3 3]
function er = lee(roll, pitch, yaw, R)

Rd = eul2rotm([yaw pitch roll], 'ZYX');

P = 1/2 * (Rd.' * R - R.' * Rd) ;

er = [P(3,2) ; P(1,3) ; P(2,1)] ;

== matlab function uas_main/quadcopter/quat 2 euler (UE) ==
  data: q input size=[1 4]; attitude output
function attitude = euler_ue(q)

attitude = quat2eul(q, 'ZYX');

attitude = [attitude(1) attitude(2) attitude(3)];

== matlab function uas_main/quadcopter/position controller/compute_roll_pitch ==
  data: F_d input; roll output; yaw_d input; pitch output
function [roll, pitch] = compute_roll_pitch(F_d, yaw_d)

yaw_dt = yaw_d + pi/2;
uyt = [cos(yaw_dt); sin(yaw_dt); 0];
uz = F_d/norm(F_d);
ux = cross(uyt, uz);
uy = cross(uz, ux);

attitude = rotm2eul([ux uy uz], 'ZYX');

roll = attitude(3);
pitch = attitude(2);

== stateflow chart uas_main/waypoint navigation (Ex. 6.1 and 7.1) ==
  state go
    pd = [r(i, 1) ; r(i, 2) ; r(i, 3)]
  (default) -> go : {i = 1}
  go -> (junction 26) : [reached(pd, p)]
  (junction 26) -> go : [i < size(r, 1)]{i = i + 1}
  data: setpoint_position function_input; position function_input; is_reached function_output; r input; i local; p input; pd output size=[3 1]
  function is_reached = reached(setpoint_position, position):
    | function is_reached = reached(setpoint_position, position)
    | is_reached = norm(position - setpoint_position) < 0.05;

== matlab function uas_main/quadcopter/quat 2 euler (ROS) ==
  data: q input size=[1 4]; roll_rad output; pitch_rad output; yaw_rad output
function [roll_rad, pitch_rad, yaw_rad] = euler_ros(q)

attitude = quat2eul(q, 'ZYX');

roll_rad = attitude(3);
pitch_rad = attitude(2);
yaw_rad = attitude(1);

== matlab function uas_main/quadcopter/MATLAB Function ==
  data: u input; y output
function y = get33(u)

y = u(3,3);
